simulink model "flood_drainage_system_2_R2025a"  (R2025a)
settings: Solver=VariableStepAuto  StartTime=0.0  StopTime=inf  FixedStep=1  RelTol=1e-3
undefined symbols (not defined in the file): DiscIntNeverNeededParam
libraries: simulink x15
(part 2 of 3)

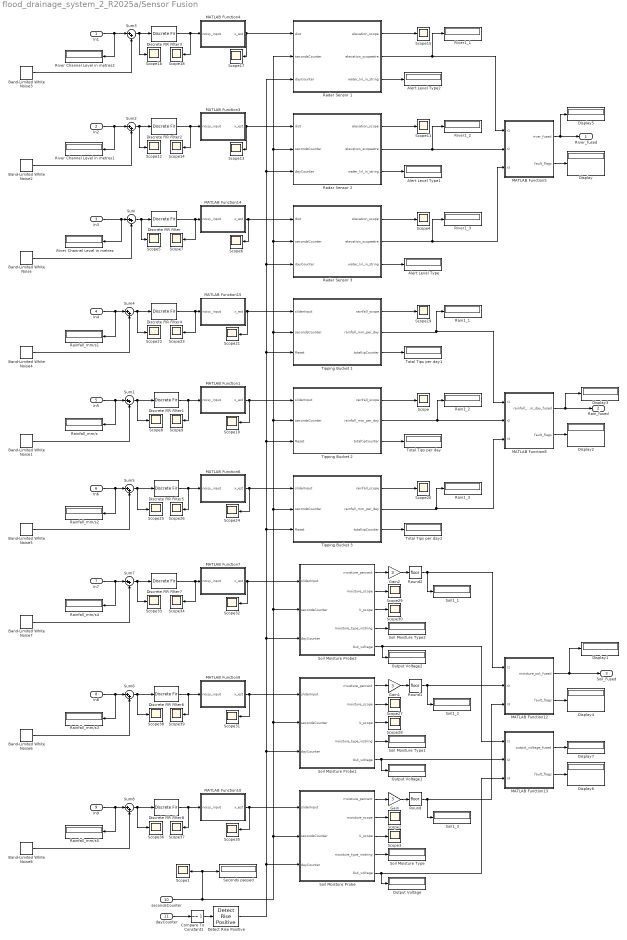
== system flood_drainage_system_2_R2025a/Sensor Fusion ==
  In1 : Inport
  In2 : Inport  Port=2
  In3 : Inport  Port=3
  In4 : Inport  Port=4
  In5 : Inport  Port=5
  In6 : Inport  Port=6
  In7 : Inport  Port=7
  In8 : Inport  Port=8
  In9 : Inport  Port=9
  secondsCounter : Inport  Port=10
  dayCounter : Inport  Port=11
  Alert Level Type : Display
  Alert Level Type1 : Display
  Alert Level Type2 : Display
  Band-Limited White Noise{,1..8} (9 alike) : simulink/Sources/Band-Limited White Noise  Cov=0.0005  Ts=1  seed=[12345]
  Compare To Constant1 : simulink/Logic and Bit Operations/Compare To Constant  relop===  const=1  OutDataTypeStr=boolean
  Detect Rise Positive : simulink/Logic and Bit Operations/Detect Rise Positive  vinit=0  OutDataTypeStr=boolean
  Discrete FIR Filter : DiscreteFir  Coefficients=[0.1 0.1 0.1 0.1 0.1 0.1 0.1 0.1 0.1 0.1]
  Discrete FIR Filter{1,4..8} (6 alike) : DiscreteFir
  Discrete FIR Filter2 : DiscreteFir  Coefficients=[0.1 0.1 0.1 0.1 0.1 0.1 0.1 0.1 0.1 0.1]
  Discrete FIR Filter3 : DiscreteFir  Coefficients=[0.1 0.1 0.1 0.1 0.1 0.1 0.1 0.1 0.1 0.1]
  Display{,1..7} (8 alike) : Display
  Gain : Gain  Gain=3
  Gain1 : Gain  Gain=3
  Gain2 : Gain  Gain=3
  MATLAB Function1 : MATLAB Function  TreatAsAtomicUnit=on
  MATLAB Function10 : MATLAB Function  TreatAsAtomicUnit=on
  MATLAB Function12 : MATLAB Function  TreatAsAtomicUnit=on
  MATLAB Function13 : MATLAB Function  TreatAsAtomicUnit=on
  MATLAB Function14 : MATLAB Function  TreatAsAtomicUnit=on
  MATLAB Function15 : MATLAB Function  TreatAsAtomicUnit=on
  MATLAB Function3 : MATLAB Function  TreatAsAtomicUnit=on
  MATLAB Function4 : MATLAB Function  TreatAsAtomicUnit=on
  MATLAB Function5 : MATLAB Function  TreatAsAtomicUnit=on
  MATLAB Function6 : MATLAB Function  TreatAsAtomicUnit=on
  MATLAB Function7 : MATLAB Function  TreatAsAtomicUnit=on
  MATLAB Function8 : MATLAB Function  TreatAsAtomicUnit=on
  MATLAB Function9 : MATLAB Function  TreatAsAtomicUnit=on
  Output Voltage : Display
  Output Voltage1 : Display
  Output Voltage2 : Display
  Radar Sensor 1 : MATLAB Function  TreatAsAtomicUnit=on
  Radar Sensor 2 : MATLAB Function  TreatAsAtomicUnit=on
  Radar Sensor 3 : MATLAB Function  TreatAsAtomicUnit=on
  Rain1_1 : Display
  Rain1_2 : Display
  Rain1_3 : Display
  Rainfall_mm/s{,1..5} (6 alike) : Display
  River Channel Level in metres : Display
  River Channel Level in metres1 : Display
  River Channel Level in metres2 : Display
  River1_1 : Display
  River1_2 : Display
  River1_3 : Display
  Round : Rounding
  Round1 : Rounding
  Round2 : Rounding
  Scope{,1..39} (40 alike) : Scope
      Scope settings: ActiveDisplayYMinimum=-10.225  ActiveDisplayYMaximum=92.025
      Scope1 settings: ActiveDisplayYMinimum=-10799.875  ActiveDisplayYMaximum=97198.875  DataLoggingVariableName=ScopeData22
      Scope10 settings: ActiveDisplayYMinimum=-0.04719  ActiveDisplayYMaximum=0.05304  DataLoggingVariableName=ScopeData23
      Scope11 settings: ActiveDisplayYMinimum=1.66242  ActiveDisplayYMaximum=5.03549  DataLoggingVariableName=ScopeData24
      Scope12 settings: ActiveDisplayYMinimum=2.1151552868576307  ActiveDisplayYMaximum=4.4405053956462046  DataLoggingVariableName=ScopeData25
      Scope13 settings: ActiveDisplayYMinimum=-1  ActiveDisplayYMaximum=1  DataLoggingVariableName=ScopeData26
      Scope14 settings: ActiveDisplayYMinimum=-1  ActiveDisplayYMaximum=1  DataLoggingVariableName=ScopeData27
      Scope15 settings: ActiveDisplayYMinimum=1.11854  ActiveDisplayYMaximum=5.0416  DataLoggingVariableName=ScopeData28
      Scope16 settings: ActiveDisplayYMinimum=3.01528  ActiveDisplayYMaximum=3.9355  DataLoggingVariableName=ScopeData29
      Scope17 settings: ActiveDisplayYMinimum=-0.04078  ActiveDisplayYMaximum=3.46295  DataLoggingVariableName=ScopeData30
      Scope18 settings: ActiveDisplayYMinimum=-0.04802  ActiveDisplayYMaximum=4.10586  DataLoggingVariableName=ScopeData31
      Scope19 settings: ActiveDisplayYMinimum=-10.225  ActiveDisplayYMaximum=92.025  DataLoggingVariableName=ScopeData32
      Scope2 settings: ActiveDisplayYMinimum=-2.30563  ActiveDisplayYMaximum=20.77423  DataLoggingVariableName=ScopeData33
      Scope20 settings: ActiveDisplayYMinimum=-10.225  ActiveDisplayYMaximum=92.025  DataLoggingVariableName=ScopeData34
      Scope21 settings: ActiveDisplayYMinimum=-0.04719  ActiveDisplayYMaximum=0.05304  DataLoggingVariableName=ScopeData35
      Scope22 settings: ActiveDisplayYMinimum=-0.13163  ActiveDisplayYMaximum=0.12145  DataLoggingVariableName=ScopeData36
      Scope23 settings: ActiveDisplayYMinimum=-0.08478  ActiveDisplayYMaximum=0.09119  DataLoggingVariableName=ScopeData5
      Scope24 settings: ActiveDisplayYMinimum=-0.04719  ActiveDisplayYMaximum=0.05304  DataLoggingVariableName=ScopeData6
      Scope25 settings: ActiveDisplayYMinimum=-0.13163  ActiveDisplayYMaximum=0.12145  DataLoggingVariableName=ScopeData7
      Scope26 settings: ActiveDisplayYMinimum=-0.08478  ActiveDisplayYMaximum=0.09119  DataLoggingVariableName=ScopeData8
      Scope27 settings: ActiveDisplayYMinimum=-3.28394  ActiveDisplayYMaximum=29.57922  DataLoggingVariableName=ScopeData9
      Scope28 settings: ActiveDisplayYMinimum=0.47959  ActiveDisplayYMaximum=0.68376  DataLoggingVariableName=ScopeData10
      Scope29 settings: ActiveDisplayYMinimum=-2.30563  ActiveDisplayYMaximum=20.77423  DataLoggingVariableName=ScopeData11
      Scope3 settings: ActiveDisplayYMinimum=0.47959  ActiveDisplayYMaximum=0.68376  DataLoggingVariableName=ScopeData37
      Scope30 settings: ActiveDisplayYMinimum=0.47959  ActiveDisplayYMaximum=0.68376  DataLoggingVariableName=ScopeData12
      Scope31 settings: ActiveDisplayYMinimum=-0.04719  ActiveDisplayYMaximum=0.05304  DataLoggingVariableName=ScopeData13
      Scope32 settings: ActiveDisplayYMinimum=-0.04719  ActiveDisplayYMaximum=0.05304  DataLoggingVariableName=ScopeData14
      Scope33 settings: ActiveDisplayYMinimum=-0.13163  ActiveDisplayYMaximum=0.12145  DataLoggingVariableName=ScopeData15
      Scope34 settings: ActiveDisplayYMinimum=-0.08478  ActiveDisplayYMaximum=0.09119  DataLoggingVariableName=ScopeData16
      Scope35 settings: ActiveDisplayYMinimum=-0.04719  ActiveDisplayYMaximum=0.05304  DataLoggingVariableName=ScopeData17
      Scope36 settings: ActiveDisplayYMinimum=-0.13163  ActiveDisplayYMaximum=0.12145  DataLoggingVariableName=ScopeData18
      Scope37 settings: ActiveDisplayYMinimum=-0.08478  ActiveDisplayYMaximum=0.09119  DataLoggingVariableName=ScopeData19
      Scope38 settings: ActiveDisplayYMinimum=-0.13163  ActiveDisplayYMaximum=0.12145  DataLoggingVariableName=ScopeData20
      Scope39 settings: ActiveDisplayYMinimum=-0.08478  ActiveDisplayYMaximum=0.09119  DataLoggingVariableName=ScopeData21
      Scope4 settings: ActiveDisplayYMinimum=2.19395  ActiveDisplayYMaximum=5.02952  DataLoggingVariableName=ScopeData4
      Scope5 settings: ActiveDisplayYMinimum=3.01528  ActiveDisplayYMaximum=3.9355  DataLoggingVariableName=ScopeData38
      Scope6 settings: ActiveDisplayYMinimum=-0.03897  ActiveDisplayYMaximum=3.3021  DataLoggingVariableName=ScopeData39
      Scope7 settings: ActiveDisplayYMinimum=-0.03899  ActiveDisplayYMaximum=3.30223  DataLoggingVariableName=ScopeData3
      Scope8 settings: ActiveDisplayYMinimum=-0.13163  ActiveDisplayYMaximum=0.12145
      Scope9 settings: ActiveDisplayYMinimum=-0.08478  ActiveDisplayYMaximum=0.09119  DataLoggingVariableName=ScopeData2
  Seconds passed : Display
  Soil Moisture Probe : MATLAB Function  TreatAsAtomicUnit=on
  Soil Moisture Probe1 : MATLAB Function  TreatAsAtomicUnit=on
  Soil Moisture Probe2 : MATLAB Function  TreatAsAtomicUnit=on
  Soil Moisture Type : Display
  Soil Moisture Type1 : Display
  Soil Moisture Type2 : Display
  Soil1_1 : Display
  Soil1_2 : Display
  Soil1_3 : Display
  Sum{,1..8} (9 alike) : Sum  Inputs=|++
  Tipping Bucket 1 : Stateflow chart  TreatAsAtomicUnit=on
      settings: PortSchema="{\"entries\":[{\"content\":{\"sides\":[{\"content\":{\"connectorIds\":[\"In1\",\"In2\",\"In3\"]},\"type\":\"ConnectorPlacement.EquallySpacedRectSide\",\"uuid\":\"5446b20b-2648-415f-9f86-c4722c72a7ab\"},{\"content\":{\"connectorIds\":[\"Out2\",\"Out3\",\"Out1\"],\"side\":\"RIGHT\"},\"type\":\"ConnectorPlacement.EquallySpacedRectSide\",\"uuid\":\"249dbc32-ec03-48ca-bf45-e180eac5a0e9\"},{\"content\":{\"side\":\"TOP\"},\"type\":\"ConnectorPlacement.EquallySpacedRectSide\",\"uuid\":\"c4af4b86-9bbe-4324-913f-65d0095b4577\"}]},\"type\":\"ConnectorPlacement.EquallySpacedConnector\",\"uuid\":\"ebffaa42-42d2-45af-8401-087243cf8eee\"}],\"packageUris\":[\"http://schema.mathworks.com/mf0/Connector/R2020b\"],\"version\":\"1.0\"}"
  Tipping Bucket 2 : Stateflow chart  TreatAsAtomicUnit=on
      settings: PortSchema="{\"entries\":[{\"content\":{\"sides\":[{\"content\":{\"connectorIds\":[\"In1\",\"In2\",\"In3\"]},\"type\":\"ConnectorPlacement.EquallySpacedRectSide\",\"uuid\":\"5446b20b-2648-415f-9f86-c4722c72a7ab\"},{\"content\":{\"connectorIds\":[\"Out2\",\"Out3\",\"Out1\"],\"side\":\"RIGHT\"},\"type\":\"ConnectorPlacement.EquallySpacedRectSide\",\"uuid\":\"249dbc32-ec03-48ca-bf45-e180eac5a0e9\"},{\"content\":{\"side\":\"TOP\"},\"type\":\"ConnectorPlacement.EquallySpacedRectSide\",\"uuid\":\"c4af4b86-9bbe-4324-913f-65d0095b4577\"}]},\"type\":\"ConnectorPlacement.EquallySpacedConnector\",\"uuid\":\"ebffaa42-42d2-45af-8401-087243cf8eee\"}],\"packageUris\":[\"http://schema.mathworks.com/mf0/Connector/R2020b\"],\"version\":\"1.0\"}"
  Tipping Bucket 3 : Stateflow chart  TreatAsAtomicUnit=on
      settings: PortSchema="{\"entries\":[{\"content\":{\"sides\":[{\"content\":{\"connectorIds\":[\"In1\",\"In2\",\"In3\"]},\"type\":\"ConnectorPlacement.EquallySpacedRectSide\",\"uuid\":\"5446b20b-2648-415f-9f86-c4722c72a7ab\"},{\"content\":{\"connectorIds\":[\"Out2\",\"Out3\",\"Out1\"],\"side\":\"RIGHT\"},\"type\":\"ConnectorPlacement.EquallySpacedRectSide\",\"uuid\":\"249dbc32-ec03-48ca-bf45-e180eac5a0e9\"},{\"content\":{\"side\":\"TOP\"},\"type\":\"ConnectorPlacement.EquallySpacedRectSide\",\"uuid\":\"c4af4b86-9bbe-4324-913f-65d0095b4577\"}]},\"type\":\"ConnectorPlacement.EquallySpacedConnector\",\"uuid\":\"ebffaa42-42d2-45af-8401-087243cf8eee\"}],\"packageUris\":[\"http://schema.mathworks.com/mf0/Connector/R2020b\"],\"version\":\"1.0\"}"
  Total Tips per day : Display
  Total Tips per day1 : Display
  Total Tips per day2 : Display
  River_fused : Outport
  Rain_fused : Outport  Port=2
  Soil_Fused : Outport  Port=3
  wires:
  Tipping Bucket 1/1(totaltipCounter) -> Total Tips per day1/1
  MATLAB Function14/1(x_est) -> Scope6/1, Radar Sensor 3/1(dist)
  Soil Moisture Probe/4(moisture_type_instring) -> Soil Moisture Type/1
  Tipping Bucket 2/3(rainfall_mm_per_day) -> MATLAB Function8/2(r2), Rain1_2/1
  MATLAB Function6/1(x_est) -> Scope24/1, Tipping Bucket 3/1(sliderInput)
  Soil Moisture Probe2/5(Out_voltage) -> MATLAB Function13/1(r1), Output Voltage2/1
  MATLAB Function13/2(fault_flags) -> Display6/1
  Sum2/1 -> Discrete FIR Filter2/1, Scope12/1
  Discrete FIR Filter8/1 -> MATLAB Function10/1(noisy_input), Scope37/1
  Discrete FIR Filter7/1 -> MATLAB Function7/1(noisy_input), Scope34/1
  Sum/1 -> Discrete FIR Filter/1, Scope5/1
  MATLAB Function8/2(fault_flags) -> Display2/1
  Tipping Bucket 3/1(totaltipCounter) -> Total Tips per day2/1
  In3/1 -> Sum/1, River Channel Level in metres/1
  Discrete FIR Filter1/1 -> MATLAB Function1/1(noisy_input), Scope9/1
  Soil Moisture Probe/1(moisture_percent) -> Gain/1
  MATLAB Function10/1(x_est) -> Soil Moisture Probe/1(sliderInput), Scope35/1
  Band-Limited White Noise5/1 -> Sum5/2
  Band-Limited White Noise8/1 -> Sum8/2
  Radar Sensor 2/1(elevation_scope) -> Scope11/1
  Sum7/1 -> Scope33/1, Discrete FIR Filter7/1
  In7/1 -> Sum7/1, Rainfall_mm/s4/1
  MATLAB Function7/1(x_est) -> Soil Moisture Probe2/1(sliderInput), Scope32/1
  In4/1 -> Sum4/1, Rainfall_mm/s1/1
  Band-Limited White Noise3/1 -> Sum3/2
  Sum1/1 -> Scope8/1, Discrete FIR Filter1/1
  Gain1/1 -> Round1/1
  secondsCounter/1 -> Seconds passed/1, Scope1/1, Soil Moisture Probe1/2(secondsCounter), Soil Moisture Probe2/2(secondsCounter), Tipping Bucket 3/2(secondsCounter), Tipping Bucket 1/2(secondsCounter), Radar Sensor 1/2(secondsCounter), Radar Sensor 2/2(secondsCounter), Radar Sensor 3/2(secondsCounter), Tipping Bucket 2/2(secondsCounter), Soil Moisture Probe/2(secondsCounter)
  Tipping Bucket 1/3(rainfall_mm_per_day) -> MATLAB Function8/1(r1), Rain1_1/1
  MATLAB Function12/2(fault_flags) -> Display4/1
  MATLAB Function9/1(x_est) -> Soil Moisture Probe1/1(sliderInput), Scope31/1
  Tipping Bucket 3/3(rainfall_mm_per_day) -> MATLAB Function8/3(r3), Rain1_3/1
  Soil Moisture Probe2/3(V_scope) -> Scope30/1
  Discrete FIR Filter6/1 -> MATLAB Function9/1(noisy_input), Scope39/1
  MATLAB Function1/1(x_est) -> Scope10/1, Tipping Bucket 2/1(sliderInput)
  Soil Moisture Probe/5(Out_voltage) -> MATLAB Function13/3(r3), Output Voltage/1
  Band-Limited White Noise/1 -> Sum/2
  Radar Sensor 1/1(elevation_scope) -> Scope15/1
  In6/1 -> Sum5/1, Rainfall_mm/s2/1
  In5/1 -> Sum1/1, Rainfall_mm/s/1
  Sum8/1 -> Scope36/1, Discrete FIR Filter8/1
  MATLAB Function8/1(rainfall_mm_day_fused) -> Display3/1, Rain_fused/1
  Radar Sensor 3/1(elevation_scope) -> Scope4/1
  Sum4/1 -> Scope22/1, Discrete FIR Filter4/1
  Tipping Bucket 2/1(totaltipCounter) -> Total Tips per day/1
  In2/1 -> Sum2/1, River Channel Level in metres1/1
  Discrete FIR Filter5/1 -> MATLAB Function6/1(noisy_input), Scope26/1
  Round1/1 -> MATLAB Function12/2(r2), Soil1_2/1
  MATLAB Function13/1(output_voltage_fused) -> Display7/1
  Radar Sensor 1/2(elevation_scopeetre) -> MATLAB Function5/1(r1), River1_1/1
  MATLAB Function4/1(x_est) -> Radar Sensor 1/1(dist), Scope17/1
  Discrete FIR Filter/1 -> Scope7/1, MATLAB Function14/1(noisy_input)
  Compare To Constant1/1 -> Detect Rise Positive/1
  Discrete FIR Filter4/1 -> MATLAB Function15/1(noisy_input), Scope23/1
  Band-Limited White Noise2/1 -> Sum2/2
  Radar Sensor 3/2(elevation_scopeetre) -> MATLAB Function5/3(r3), River1_3/1
  Round/1 -> Soil1_3/1, MATLAB Function12/3(r3)
  Detect Rise Positive/1 -> Soil Moisture Probe1/3(dayCounter), Soil Moisture Probe2/3(dayCounter), Tipping Bucket 3/3(Reset), Tipping Bucket 1/3(Reset), Radar Sensor 1/3(dayCounter), Radar Sensor 2/3(dayCounter), Radar Sensor 3/3(dayCounter), Tipping Bucket 2/3(Reset), Soil Moisture Probe/3(dayCounter)
  MATLAB Function15/1(x_est) -> Scope21/1, Tipping Bucket 1/1(sliderInput)
  Sum3/1 -> Discrete FIR Filter3/1, Scope16/1
  In8/1 -> Sum6/1, Rainfall_mm/s3/1
  Gain/1 -> Round/1
  MATLAB Function5/1(river_fused) -> Display5/1, River_fused/1
  Soil Moisture Probe1/2(moisture_scope) -> Scope27/1
  Discrete FIR Filter3/1 -> Scope18/1, MATLAB Function4/1(noisy_input)
  Soil Moisture Probe2/4(moisture_type_instring) -> Soil Moisture Type2/1
  Radar Sensor 3/3(water_lvl_in_string) -> Alert Level Type/1
  MATLAB Function3/1(x_est) -> Radar Sensor 2/1(dist), Scope13/1
  Sum6/1 -> Scope38/1, Discrete FIR Filter6/1
  Soil Moisture Probe1/3(V_scope) -> Scope28/1
  Soil Moisture Probe/3(V_scope) -> Scope3/1
  Tipping Bucket 1/2(rainfall_scope) -> Scope19/1
  Band-Limited White Noise4/1 -> Sum4/2
  Discrete FIR Filter2/1 -> MATLAB Function3/1(noisy_input), Scope14/1
  Band-Limited White Noise7/1 -> Sum7/2
  Round2/1 -> MATLAB Function12/1(r1), Soil1_1/1
  MATLAB Function5/2(fault_flags) -> Display/1
  Gain2/1 -> Round2/1
  Soil Moisture Probe2/1(moisture_percent) -> Gain2/1
  Tipping Bucket 2/2(rainfall_scope) -> Scope/1
  Radar Sensor 2/3(water_lvl_in_string) -> Alert Level Type1/1
  Soil Moisture Probe2/2(moisture_scope) -> Scope29/1
  In9/1 -> Sum8/1, Rainfall_mm/s5/1
  Soil Moisture Probe1/1(moisture_percent) -> Gain1/1
  Radar Sensor 2/2(elevation_scopeetre) -> River1_2/1, MATLAB Function5/2(r2)
  Soil Moisture Probe/2(moisture_scope) -> Scope2/1
  Sum5/1 -> Scope25/1, Discrete FIR Filter5/1
  Radar Sensor 1/3(water_lvl_in_string) -> Alert Level Type2/1
  Band-Limited White Noise6/1 -> Sum6/2
  Band-Limited White Noise1/1 -> Sum1/2
  Soil Moisture Probe1/5(Out_voltage) -> MATLAB Function13/2(r2), Output Voltage1/1
  Soil Moisture Probe1/4(moisture_type_instring) -> Soil Moisture Type1/1
  In1/1 -> Sum3/1, River Channel Level in metres2/1
  MATLAB Function12/1(moisture_pct_fused) -> Display1/1, Soil_Fused/1
  Tipping Bucket 3/2(rainfall_scope) -> Scope20/1
  dayCounter/1 -> Compare To Constant1/1

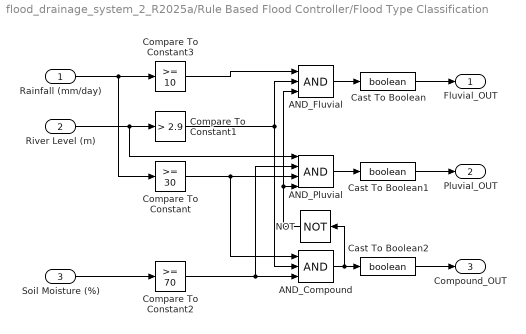
== system flood_drainage_system_2_R2025a/Rule Based Flood Controller/Flood Type Classification ==
  Rainfall (mm/day) : Inport
  River Level (m) : Inport  Port=2
  Soil Moisture (%) : Inport  Port=3
  AND_Compound : Logic  Inputs=3  IconShape=distinctive  AllPortsSameDT=off  OutDataTypeStr=boolean
  AND_Fluvial : Logic  Inputs=3  IconShape=distinctive  AllPortsSameDT=off  OutDataTypeStr=boolean
  AND_Pluvial : Logic  Inputs=4  IconShape=distinctive  AllPortsSameDT=off  OutDataTypeStr=boolean
  Cast To Boolean : DataTypeConversion  OutDataTypeStr=boolean  SaturateOnIntegerOverflow=off  RndMeth=Floor
  Cast To Boolean1 : DataTypeConversion  OutDataTypeStr=boolean  SaturateOnIntegerOverflow=off  RndMeth=Floor
  Cast To Boolean2 : DataTypeConversion  OutDataTypeStr=boolean  SaturateOnIntegerOverflow=off  RndMeth=Floor
  Compare To Constant : simulink/Logic and Bit Operations/Compare To Constant  relop=>=  const=30  OutDataTypeStr=boolean
  Compare To Constant1 : simulink/Logic and Bit Operations/Compare To Constant  relop=>  const=2.9  OutDataTypeStr=boolean
  Compare To Constant2 : simulink/Logic and Bit Operations/Compare To Constant  relop=>=  const=70  OutDataTypeStr=boolean
  Compare To Constant3 : simulink/Logic and Bit Operations/Compare To Constant  relop=>=  const=10  OutDataTypeStr=boolean
  NOT : Logic  Operator=NOT  IconShape=distinctive  AllPortsSameDT=off  OutDataTypeStr=boolean
  Fluvial_OUT : Outport
  Pluvial_OUT : Outport  Port=2
  Compound_OUT : Outport  Port=3
  wires:
  Rainfall (mm/day)/1 -> Compare To Constant/1, Compare To Constant3/1
  River Level (m)/1 -> AND_Pluvial/1, Compare To Constant1/1
  Soil Moisture (%)/1 -> Compare To Constant2/1
  Compare To Constant/1 -> AND_Compound/1, AND_Pluvial/3
  Compare To Constant1/1 -> AND_Fluvial/2, AND_Compound/2
  Compare To Constant2/1 -> AND_Pluvial/2, AND_Compound/3
  Compare To Constant3/1 -> AND_Fluvial/1
  AND_Fluvial/1 -> Cast To Boolean/1
  Cast To Boolean/1 -> Fluvial_OUT/1
  Cast To Boolean1/1 -> Pluvial_OUT/1
  AND_Compound/1 -> NOT/1, Cast To Boolean2/1
  AND_Pluvial/1 -> Cast To Boolean1/1
  Cast To Boolean2/1 -> Compound_OUT/1
  NOT/1 -> AND_Fluvial/3, AND_Pluvial/4

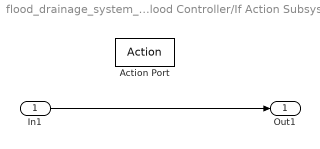
== system flood_drainage_system_2_R2025a/Rule Based Flood Controller/If Action Subsystem ==
  In1 : Inport
  Action Port : ActionPort  ActionPortLabel=if(u1 <= 0.3)
  Out1 : Outport
  wires:
  In1/1 -> Out1/1

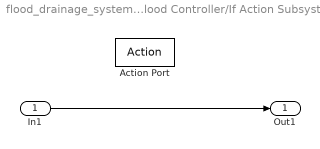
== system flood_drainage_system_2_R2025a/Rule Based Flood Controller/If Action Subsystem1 ==
  In1 : Inport
  Action Port : ActionPort  ActionPortLabel=elseif(u1 <= 0.6)
  Out1 : Outport
  wires:
  In1/1 -> Out1/1

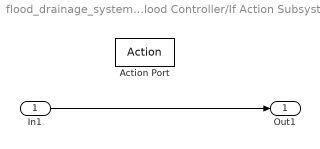
== system flood_drainage_system_2_R2025a/Rule Based Flood Controller/If Action Subsystem2 ==
  In1 : Inport
  Action Port : ActionPort  ActionPortLabel=elseif(u1 < 0.8)
  Out1 : Outport
  wires:
  In1/1 -> Out1/1

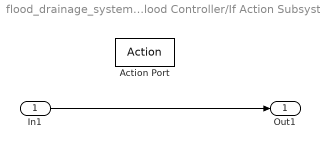
== system flood_drainage_system_2_R2025a/Rule Based Flood Controller/If Action Subsystem3 ==
  In1 : Inport
  Action Port : ActionPort  ActionPortLabel=else
  Out1 : Outport
  wires:
  In1/1 -> Out1/1

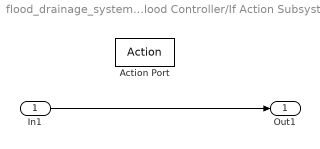
== system flood_drainage_system_2_R2025a/Rule Based Flood Controller/If Action Subsystem4 ==
  In1 : Inport
  Action Port : ActionPort  ActionPortLabel=if(u1==1)
  Out1 : Outport
  wires:
  In1/1 -> Out1/1

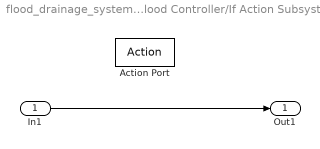
== system flood_drainage_system_2_R2025a/Rule Based Flood Controller/If Action Subsystem5 ==
  In1 : Inport
  Action Port : ActionPort  ActionPortLabel=elseif(u1==2)
  Out1 : Outport
  wires:
  In1/1 -> Out1/1

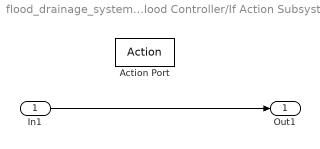
== system flood_drainage_system_2_R2025a/Rule Based Flood Controller/If Action Subsystem6 ==
  In1 : Inport
  Action Port : ActionPort  ActionPortLabel=elseif(u1==3)
  Out1 : Outport
  wires:
  In1/1 -> Out1/1

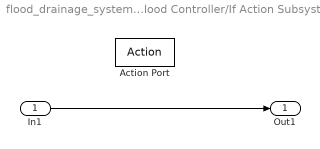
== system flood_drainage_system_2_R2025a/Rule Based Flood Controller/If Action Subsystem7 ==
  In1 : Inport
  Action Port : ActionPort  ActionPortLabel=else
  Out1 : Outport
  wires:
  In1/1 -> Out1/1

== matlab function flood_drainage_system_2_R2025a/Sensor Fusion/Radar Sensor 2 ==
  data: dist input; elevation_scope output; secondsCounter input; dayCounter input; elevation_scopeetre output; water_lvl_in_string output
function [elevation_scope, elevation_scopeetre, water_lvl_in_string] = ...
          riverElevationSensor(dist, secondsCounter, dayCounter)

ref_elev = 5.0; % reference elevation (m)

persistent prevSec prevDay elevation elevation_last water_lvl_code_last water_lvl_str_last
if isempty(prevSec), prevSec = 0; end
if isempty(prevDay), prevDay = 0; end
if isempty(elevation), elevation = ref_elev - dist; end
if isempty(elevation_last), elevation_last = ref_elev - dist; end
if isempty(water_lvl_code_last), water_lvl_code_last = 0; end
if isempty(water_lvl_str_last), water_lvl_str_last = "Error"; end

deltaT = secondsCounter - prevSec;
if deltaT <= 0
    deltaT = 1;
end

% update elevation by the second
target_elev = ref_elev - dist;
rate = (target_elev - elevation) / 1000; % smoothing factor
elevation = elevation + rate * deltaT;

% classification
% If elevation_scope is higher than:
% 1.7 m = Critical
% 2.05 m = Alert
% 2.2 m = Normal

if elevation > 2.05 % Below 2.05 m = Normal
    water_lvl_code = 1; % Normal
    water_lvl_str = "Normal";
elseif (elevation <= 2.05 && elevation > 1.7)
    water_lvl_code = 2; % Alert
    water_lvl_str = "Alert";
elseif elevation <= 1.7 
    water_lvl_code = 3; % Critical
    water_lvl_str = "Critical";
else
    water_lvl_code = 0; % Error
    water_lvl_str = "Error";
end

% reset logic
if double(dayCounter) ~= double(prevDay)
    elevation_last = elevation;
    water_lvl_code_last = water_lvl_code;
    water_lvl_str_last = water_lvl_str;
    prevDay = double(dayCounter);
end

% update state
prevSec = secondsCounter;

% outputs
elevation_scope = elevation;
elevation_scopeetre = elevation_last;
water_lvl_in_string = water_lvl_str_last;

== matlab function flood_drainage_system_2_R2025a/MATLAB Function2 ==
  data: secondsCounter output; dayCounter output; u input
function [secondsCounter, dayCounter] = timerFcn(u)

persistent seconds day
if isempty(seconds)
    seconds = 0;
end

if isempty(day)
    day = 0;
end

% count seconds to full day
seconds = seconds + 1;

% full day passed (24 hours = 86400 sec)
if mod(seconds,86400 ) == 0
    day = day + 1;
end

% output
secondsCounter = mod(seconds,86400);
dayCounter = day;

== matlab function flood_drainage_system_2_R2025a/Sensor Fusion/Soil Moisture Probe ==
  data: moisture_percent output; moisture_scope output; V_scope output; sliderInput input; secondsCounter input; dayCounter input; moisture_type_instring output; Out_voltage output
function [moisture_percent, moisture_scope, V_scope, moisture_type_instring, Out_voltage] = ...
          soilMoistureProbe(sliderInput, secondsCounter, dayCounter)

infil_eff = 0.7;       % infiltration efficiency
d = 300;               % soil depth (mm)
ET_day = 2;            % evapotranspiration loss (mm/day)
ET_rate = ET_day / 86400; % mm/s

persistent VWC prevSec prevDay moisture_scope_last moisture_type_last V_scope_last
if isempty(VWC), VWC = 0; end
if isempty(prevSec), prevSec = 0; end
if isempty(prevDay), prevDay = 0; end
if isempty(moisture_scope_last), moisture_scope_last = 0; end
if isempty(moisture_type_last), moisture_type_last = ""; end
if isempty(V_scope_last), V_scope_last = 0; end

% deltaT (seconds since last tick)
deltaT = secondsCounter - prevSec;
if deltaT <= 0
    deltaT = 1;
end

% rainfall over deltaT (per sec)
rain_mm = sliderInput * deltaT;          % mm of rain in deltaT (per sec)
infil_mm = infil_eff * rain_mm;          % effective infiltration
rain_frac = infil_mm / d;                % fraction of saturation

% ET contribution over deltaT
ET_mm = ET_rate * deltaT;                % mm lost in deltaT
ET_frac = ET_mm / d;                     % fraction of saturation

% Update cumulative Volume Water Concentration (VWC) in fraction
VWC = VWC + rain_frac - ET_frac;
moisture_scope = VWC * 100;

% keep between 0 to 100 only
moisture_scope = max(0, min(100, moisture_scope));
VWC = moisture_scope / 100; 

% classification
if  moisture_scope < 10 % 30
    moisture_type = "Dry";
elseif moisture_scope < 20 % 60
    moisture_type = "Moderate";
elseif moisture_scope < 30 % 90
    moisture_type = "Wet";
else
    moisture_type = "Saturated";
end

% voltage output
V_scope = 0.5 + (moisture_scope/100);

% reset logic (daily rollover)
if double(dayCounter) ~= double(prevDay)
    moisture_scope_last = moisture_scope;
    moisture_type_last = moisture_type;
    V_scope_last = V_scope;

    % carry forward baseline
    VWC = moisture_scope / 100;
    prevDay = double(dayCounter);
end

% update state
prevSec = secondsCounter;

% outputs
moisture_percent = moisture_scope_last;
moisture_type_instring = moisture_type_last;
Out_voltage = V_scope_last;

== matlab function flood_drainage_system_2_R2025a/Sensor Fusion/Radar Sensor 3 ==
  data: dist input; elevation_scope output; secondsCounter input; dayCounter input; elevation_scopeetre output; water_lvl_in_string output
function [elevation_scope, elevation_scopeetre, water_lvl_in_string] = ...
          riverElevationSensor(dist, secondsCounter, dayCounter)

ref_elev = 5.0; % reference elevation (m)

persistent prevSec prevDay elevation elevation_last water_lvl_code_last water_lvl_str_last
if isempty(prevSec), prevSec = 0; end
if isempty(prevDay), prevDay = 0; end
if isempty(elevation), elevation = ref_elev - dist; end
if isempty(elevation_last), elevation_last = ref_elev - dist; end
if isempty(water_lvl_code_last), water_lvl_code_last = 0; end
if isempty(water_lvl_str_last), water_lvl_str_last = "Error"; end

deltaT = secondsCounter - prevSec;
if deltaT <= 0
    deltaT = 1;
end

% update elevation by the second
target_elev = ref_elev - dist;
rate = (target_elev - elevation) / 1000; % smoothing factor
elevation = elevation + rate * deltaT;

% classification
% If elevation_scope is higher than:
% 1.7 m = Critical
% 2.05 m = Alert
% 2.2 m = Normal

if elevation > 2.05 % Below 2.05 m = Normal
    water_lvl_code = 1; % Normal
    water_lvl_str = "Normal";
elseif (elevation <= 2.05 && elevation > 1.7)
    water_lvl_code = 2; % Alert
    water_lvl_str = "Alert";
elseif elevation <= 1.7 
    water_lvl_code = 3; % Critical
    water_lvl_str = "Critical";
else
    water_lvl_code = 0; % Error
    water_lvl_str = "Error";
end

% reset logic
if double(dayCounter) ~= double(prevDay)
    elevation_last = elevation;
    water_lvl_code_last = water_lvl_code;
    water_lvl_str_last = water_lvl_str;
    prevDay = double(dayCounter);
end

% update state
prevSec = secondsCounter;

% outputs
elevation_scope = elevation;
elevation_scopeetre = elevation_last;
water_lvl_in_string = water_lvl_str_last;

== matlab function flood_drainage_system_2_R2025a/Sensor Fusion/MATLAB Function4 ==
  data: noisy_input input; x_est output
function x_est = kalmanFilter(noisy_input)

persistent x P
if isempty(x), x = noisy_input; end
if isempty(P), P = 1; end


Q = 1e-3;   % process noise covariance
R = 1e-4;   % measurement noise covariance

% prediction
x_pred = x;
P_pred = P + Q;

% update
K = P_pred / (P_pred + R);
x = x_pred + K*(noisy_input - x_pred);
P = (1 - K)*P_pred;

x_est = x;

== matlab function flood_drainage_system_2_R2025a/Sensor Fusion/Radar Sensor 1 ==
  data: dist input; elevation_scope output; secondsCounter input; dayCounter input; elevation_scopeetre output; water_lvl_in_string output
function [elevation_scope, elevation_scopeetre, water_lvl_in_string] = ...
          riverElevationSensor(dist, secondsCounter, dayCounter)

ref_elev = 5.0; % reference elevation (m)

persistent prevSec prevDay elevation elevation_last water_lvl_code_last water_lvl_str_last
if isempty(prevSec), prevSec = 0; end
if isempty(prevDay), prevDay = 0; end
if isempty(elevation), elevation = ref_elev - dist; end
if isempty(elevation_last), elevation_last = ref_elev - dist; end
if isempty(water_lvl_code_last), water_lvl_code_last = 0; end
if isempty(water_lvl_str_last), water_lvl_str_last = "Error"; end

deltaT = secondsCounter - prevSec;
if deltaT <= 0
    deltaT = 1;
end

% update elevation by the second
target_elev = ref_elev - dist;
rate = (target_elev - elevation) / 1000; % smoothing factor
elevation = elevation + rate * deltaT;

% classification
% If elevation_scope is higher than:
% 1.7 m = Critical
% 2.05 m = Alert
% 2.2 m = Normal

if elevation > 2.05 % Below 2.05 m = Normal
    water_lvl_code = 1; % Normal
    water_lvl_str = "Normal";
elseif (elevation <= 2.05 && elevation > 1.7)
    water_lvl_code = 2; % Alert
    water_lvl_str = "Alert";
elseif elevation <= 1.7 
    water_lvl_code = 3; % Critical
    water_lvl_str = "Critical";
else
    water_lvl_code = 0; % Error
    water_lvl_str = "Error";
end

% reset logic
if double(dayCounter) ~= double(prevDay)
    elevation_last = elevation;
    water_lvl_code_last = water_lvl_code;
    water_lvl_str_last = water_lvl_str;
    prevDay = double(dayCounter);
end

% update state
prevSec = secondsCounter;

% outputs
elevation_scope = elevation;
elevation_scopeetre = elevation_last;
water_lvl_in_string = water_lvl_str_last;

== matlab function flood_drainage_system_2_R2025a/Sensor Fusion/MATLAB Function5 ==
  data: r1 input; river_fused output; r2 input; r3 input; fault_flags output
function [river_fused, fault_flags] = fuseRiverSensors(r1, r2, r3)
% r1, r2, r3 = filtered outputs from 3 sensor chains
% river_fused = fused river elevation signal (scalar double)
% fault_flags = [f1 f2 f3], 1 if sensor flagged faulty

% Parameters
tol = 0.10; % 10% tolerance

% Step 1: Compute mean
vals = [r1 r2 r3];
mean_val = mean(vals);

% Step 2: Fault detection
fault_flags = abs(vals - mean_val) > tol*mean_val;

% Step 3: Fuse valid sensors
valid_vals = vals(~fault_flags);

if isempty(valid_vals)
    % All faulty → fallback to mean
    river_fused = mean_val;
elseif isscalar(valid_vals)
    % Only one valid → use it directly (scalar)
    river_fused = valid_vals(1);
elseif numel(valid_vals) == 2
    % Two valid → average them (scalar)
    river_fused = mean(valid_vals);
else
    % All valid (3) → use median (scalar)
    river_fused = median(valid_vals);
end

== stateflow chart flood_drainage_system_2_R2025a/Sensor Fusion/Tipping Bucket 1 ==
  state Collecting
    during:
    [accumulation, tipCounter, rainfall_scope] = bucketMath(sliderInput, secondsCounter);
  state Reset_Signal
    entry:
    rainfall_mm_per_day = rainfall_scope;
    totaltipCounter = tipCounter;
    tipCounter = 0;
    accumulation = 0;
    rainfall_scope = 0;
  (default) -> Collecting
  Reset_Signal -> Collecting
  Collecting -> Reset_Signal : [Reset == 1]
  data: sliderInput function_input; accumulation function_output; tipCounter function_output; rainfall_scope function_output; secondsCounter function_input; totaltipCounter output; rainfall_scope output; sliderInput input; accumulation local; secondsCounter input; Reset input; rainfall_mm_per_day output; tipCounter local
  function [accumulation, tipCounter, rainfall_scope] = bucketMath(sliderInput, secondsCounter):
    | function [accumulation, tipCounter, rainfall_scope] = bucketMath(sliderInput, secondsCounter)
    | 
    | persistent acc tips prevSec
    | if isempty(acc), acc = 0; end
    | if isempty(tips), tips = 0; end
    | if isempty(prevSec), prevSec = 0; end
    | 
    | deltaT = secondsCounter - prevSec;
    | if deltaT <= 0, deltaT = 1; end
    | 
    | acc = acc + sliderInput * deltaT;
    | if acc >= 0.2
    |     tips = tips + 1;
    |     acc = acc - 0.2;
    | end
    | 
    | rainfall_scope = tips * 0.2;
    | prevSec = secondsCounter;
    | 
    | accumulation = acc;
    | tipCounter = tips;

== stateflow chart flood_drainage_system_2_R2025a/Sensor Fusion/Tipping Bucket 2 ==
  state Collecting
    during:
    [accumulation, tipCounter, rainfall_scope] = bucketMath(sliderInput, secondsCounter);
  state Reset_Signal
    entry:
    rainfall_mm_per_day = rainfall_scope;
    totaltipCounter = tipCounter;
    tipCounter = 0;
    accumulation = 0;
    rainfall_scope = 0;
  (default) -> Collecting
  Reset_Signal -> Collecting
  Collecting -> Reset_Signal : [Reset == 1]
  data: sliderInput function_input; accumulation function_output; tipCounter function_output; rainfall_scope function_output; secondsCounter function_input; totaltipCounter output; rainfall_scope output; sliderInput input; accumulation local; secondsCounter input; Reset input; rainfall_mm_per_day output; tipCounter local
  function [accumulation, tipCounter, rainfall_scope] = bucketMath(sliderInput, secondsCounter):
    | function [accumulation, tipCounter, rainfall_scope] = bucketMath(sliderInput, secondsCounter)
    | persistent acc tips prevSec
    | if isempty(acc), acc = 0; end
    | if isempty(tips), tips = 0; end
    | if isempty(prevSec), prevSec = 0; end
    | 
    | deltaT = secondsCounter - prevSec;
    | if deltaT <= 0, deltaT = 1; end
    | 
    | acc = acc + sliderInput * deltaT;
    | if acc >= 0.2
    |     tips = tips + 1;
    |     acc = acc - 0.2;
    | end
    | 
    | rainfall_scope = tips * 0.2;
    | prevSec = secondsCounter;
    | 
    | accumulation = acc;
    | tipCounter = tips;

== matlab function flood_drainage_system_2_R2025a/Sensor Fusion/MATLAB Function6 ==
  data: noisy_input input; x_est output
function x_est = kalmanFilter(noisy_input)

persistent x P
if isempty(x), x = noisy_input; end
if isempty(P), P = 1; end


Q = 1e-3;   % process noise covariance
R = 1e-4;   % measurement noise covariance

% prediction
x_pred = x;
P_pred = P + Q;

% update
K = P_pred / (P_pred + R);
x = x_pred + K*(noisy_input - x_pred);
P = (1 - K)*P_pred;

x_est = x;

== matlab function flood_drainage_system_2_R2025a/Sensor Fusion/MATLAB Function7 ==
  data: noisy_input input; x_est output
function x_est = kalmanFilter(noisy_input)

persistent x P
if isempty(x), x = noisy_input; end
if isempty(P), P = 1; end


Q = 1e-3;   % process noise covariance
R = 1e-4;   % measurement noise covariance

% prediction
x_pred = x;
P_pred = P + Q;

% update
K = P_pred / (P_pred + R);
x = x_pred + K*(noisy_input - x_pred);
P = (1 - K)*P_pred;

x_est = x;

== matlab function flood_drainage_system_2_R2025a/Sensor Fusion/MATLAB Function8 ==
  data: r1 input; rainfall_mm_day_fused output; r2 input; r3 input; fault_flags output
function [rainfall_mm_day_fused, fault_flags] = fuseTipBucSensors(r1, r2, r3)
% r1, r2, r3 = filtered outputs from 3 sensor chains
% rainfall_mm_day_fused = fused river elevation signal (scalar double)
% fault_flags = [f1 f2 f3], 1 if sensor flagged faulty

% Parameters
tol = 0.15; % 15% tolerance

% Step 1: Compute mean
vals = [r1 r2 r3];
mean_val = mean(vals);

% Step 2: Fault detection
fault_flags = abs(vals - mean_val) > tol*mean_val;

% Step 3: Fuse valid sensors
valid_vals = vals(~fault_flags);

if isempty(valid_vals)
    % All faulty → fallback to mean
    rainfall_mm_day_fused = mean_val;
elseif isscalar(valid_vals)
    % Only one valid → use it directly (scalar)
    rainfall_mm_day_fused = valid_vals(1);
elseif numel(valid_vals) == 2
    % Two valid → average them (scalar)
    rainfall_mm_day_fused = mean(valid_vals);
else
    % All valid (3) → use median (scalar)
    rainfall_mm_day_fused = median(valid_vals);
end

== matlab function flood_drainage_system_2_R2025a/Sensor Fusion/Soil Moisture Probe1 ==
  data: moisture_percent output; moisture_scope output; V_scope output; sliderInput input; secondsCounter input; dayCounter input; moisture_type_instring output; Out_voltage output
function [moisture_percent, moisture_scope, V_scope, moisture_type_instring, Out_voltage] = ...
          soilMoistureProbe(sliderInput, secondsCounter, dayCounter)

infil_eff = 0.7;       % infiltration efficiency
d = 300;               % soil depth (mm)
ET_day = 2;            % evapotranspiration loss (mm/day)
ET_rate = ET_day / 86400; % mm/s

persistent VWC prevSec prevDay moisture_scope_last moisture_type_last V_scope_last
if isempty(VWC), VWC = 0; end
if isempty(prevSec), prevSec = 0; end
if isempty(prevDay), prevDay = 0; end
if isempty(moisture_scope_last), moisture_scope_last = 0; end
if isempty(moisture_type_last), moisture_type_last = ""; end
if isempty(V_scope_last), V_scope_last = 0; end

% deltaT (seconds since last tick)
deltaT = secondsCounter - prevSec;
if deltaT <= 0
    deltaT = 1;
end

% rainfall over deltaT (per sec)
rain_mm = sliderInput * deltaT;          % mm of rain in deltaT (per sec)
infil_mm = infil_eff * rain_mm;          % effective infiltration
rain_frac = infil_mm / d;                % fraction of saturation

% ET contribution over deltaT
ET_mm = ET_rate * deltaT;                % mm lost in deltaT
ET_frac = ET_mm / d;                     % fraction of saturation

% Update cumulative Volume Water Concentration (VWC) in fraction
VWC = VWC + rain_frac - ET_frac;
moisture_scope = VWC * 100;

% keep between 0 to 100 only
moisture_scope = max(0, min(100, moisture_scope));
VWC = moisture_scope / 100; 

% classification
if  moisture_scope < 10 % 30
    moisture_type = "Dry";
elseif moisture_scope < 20 % 60
    moisture_type = "Moderate";
elseif moisture_scope < 30 % 90
    moisture_type = "Wet";
else
    moisture_type = "Saturated";
end

% voltage output
V_scope = 0.5 + (moisture_scope/100);

% reset logic (daily rollover)
if double(dayCounter) ~= double(prevDay)
    moisture_scope_last = moisture_scope;
    moisture_type_last = moisture_type;
    V_scope_last = V_scope;

    % carry forward baseline
    VWC = moisture_scope / 100;
    prevDay = double(dayCounter);
end

% update state
prevSec = secondsCounter;

% outputs
moisture_percent = moisture_scope_last;
moisture_type_instring = moisture_type_last;
Out_voltage = V_scope_last;

== matlab function flood_drainage_system_2_R2025a/Sensor Fusion/Soil Moisture Probe2 ==
  data: moisture_percent output; moisture_scope output; V_scope output; sliderInput input; secondsCounter input; dayCounter input; moisture_type_instring output; Out_voltage output
function [moisture_percent, moisture_scope, V_scope, moisture_type_instring, Out_voltage] = ...
          soilMoistureProbe(sliderInput, secondsCounter, dayCounter)

infil_eff = 0.7;       % infiltration efficiency
d = 300;               % soil depth (mm)
ET_day = 2;            % evapotranspiration loss (mm/day)
ET_rate = ET_day / 86400; % mm/s

persistent VWC prevSec prevDay moisture_scope_last moisture_type_last V_scope_last
if isempty(VWC), VWC = 0; end
if isempty(prevSec), prevSec = 0; end
if isempty(prevDay), prevDay = 0; end
if isempty(moisture_scope_last), moisture_scope_last = 0; end
if isempty(moisture_type_last), moisture_type_last = ""; end
if isempty(V_scope_last), V_scope_last = 0; end

% deltaT (seconds since last tick)
deltaT = secondsCounter - prevSec;
if deltaT <= 0
    deltaT = 1;
end

% rainfall over deltaT (per sec)
rain_mm = sliderInput * deltaT;          % mm of rain in deltaT (per sec)
infil_mm = infil_eff * rain_mm;          % effective infiltration
rain_frac = infil_mm / d;                % fraction of saturation

% ET contribution over deltaT
ET_mm = ET_rate * deltaT;                % mm lost in deltaT
ET_frac = ET_mm / d;                     % fraction of saturation

% Update cumulative Volume Water Concentration (VWC) in fraction
VWC = VWC + rain_frac - ET_frac;
moisture_scope = VWC * 100;

% keep between 0 to 100 only
moisture_scope = max(0, min(100, moisture_scope));
VWC = moisture_scope / 100; 

% classification
if  moisture_scope < 10 % 30
    moisture_type = "Dry";
elseif moisture_scope < 20 % 60
    moisture_type = "Moderate";
elseif moisture_scope < 30 % 90
    moisture_type = "Wet";
else
    moisture_type = "Saturated";
end

% voltage output
V_scope = 0.5 + (moisture_scope/100);

% reset logic (daily rollover)
if double(dayCounter) ~= double(prevDay)
    moisture_scope_last = moisture_scope;
    moisture_type_last = moisture_type;
    V_scope_last = V_scope;

    % carry forward baseline
    VWC = moisture_scope / 100;
    prevDay = double(dayCounter);
end

% update state
prevSec = secondsCounter;

% outputs
moisture_percent = moisture_scope_last;
moisture_type_instring = moisture_type_last;
Out_voltage = V_scope_last;

== matlab function flood_drainage_system_2_R2025a/Sensor Fusion/MATLAB Function9 ==
  data: noisy_input input; x_est output
function x_est = kalmanFilter(noisy_input)

persistent x P
if isempty(x), x = noisy_input; end
if isempty(P), P = 1; end


Q = 1e-3;   % process noise covariance
R = 1e-4;   % measurement noise covariance

% prediction
x_pred = x;
P_pred = P + Q;

% update
K = P_pred / (P_pred + R);
x = x_pred + K*(noisy_input - x_pred);
P = (1 - K)*P_pred;

x_est = x;

== matlab function flood_drainage_system_2_R2025a/Sensor Fusion/MATLAB Function10 ==
  data: noisy_input input; x_est output
function x_est = kalmanFilter(noisy_input)

persistent x P
if isempty(x), x = noisy_input; end
if isempty(P), P = 1; end


Q = 1e-3;   % process noise covariance
R = 1e-4;   % measurement noise covariance

% prediction
x_pred = x;
P_pred = P + Q;

% update
K = P_pred / (P_pred + R);
x = x_pred + K*(noisy_input - x_pred);
P = (1 - K)*P_pred;

x_est = x;

== stateflow chart flood_drainage_system_2_R2025a/Sensor Fusion/Tipping Bucket 3 ==
  state Collecting
    during:
    [accumulation, tipCounter, rainfall_scope] = bucketMath(sliderInput, secondsCounter);
  state Reset_Signal
    entry:
    rainfall_mm_per_day = rainfall_scope;
    totaltipCounter = tipCounter;
    tipCounter = 0;
    accumulation = 0;
    rainfall_scope = 0;
  (default) -> Collecting
  Reset_Signal -> Collecting
  Collecting -> Reset_Signal : [Reset == 1]
  data: sliderInput function_input; accumulation function_output; tipCounter function_output; rainfall_scope function_output; secondsCounter function_input; totaltipCounter output; rainfall_scope output; sliderInput input; accumulation local; secondsCounter input; Reset input; rainfall_mm_per_day output; tipCounter local
  function [accumulation, tipCounter, rainfall_scope] = bucketMath(sliderInput, secondsCounter):
    | function [accumulation, tipCounter, rainfall_scope] = bucketMath(sliderInput, secondsCounter)
    | persistent acc tips prevSec
    | if isempty(acc), acc = 0; end
    | if isempty(tips), tips = 0; end
    | if isempty(prevSec), prevSec = 0; end
    | 
    | deltaT = secondsCounter - prevSec;
    | if deltaT <= 0, deltaT = 1; end
    | 
    | acc = acc + sliderInput * deltaT;
    | if acc >= 0.2
    |     tips = tips + 1;
    |     acc = acc - 0.2;
    | end
    | 
    | rainfall_scope = tips * 0.2;
    | prevSec = secondsCounter;
    | 
    | accumulation = acc;
    | tipCounter = tips;

== matlab function flood_drainage_system_2_R2025a/Sensor Fusion/MATLAB Function12 ==
  data: r1 input; moisture_pct_fused output; r2 input; r3 input; fault_flags output
function [moisture_pct_fused, fault_flags] = fuseSoilMoistSensors(r1, r2, r3)
% r1, r2, r3 = filtered outputs from 3 sensor chains
% moisture_pct_fused = fused river elevation signal (scalar double)
% fault_flags = [f1 f2 f3], 1 if sensor flagged faulty

% Parameters
tol = 0.13; % 13% tolerance

% Step 1: Compute mean
vals = [r1 r2 r3];
mean_val = mean(vals);

% Step 2: Fault detection
fault_flags = abs(vals - mean_val) > tol*mean_val;

% Step 3: Fuse valid sensors
valid_vals = vals(~fault_flags);

if isempty(valid_vals)
    % All faulty → fallback to mean
    moisture_pct_fused = mean_val;
elseif isscalar(valid_vals)
    % Only one valid → use it directly (scalar)
    moisture_pct_fused = valid_vals(1);
elseif numel(valid_vals) == 2
    % Two valid → average them (scalar)
    moisture_pct_fused = mean(valid_vals);
else
    % All valid (3) → use median (scalar)
    moisture_pct_fused = median(valid_vals);
end

== matlab function flood_drainage_system_2_R2025a/Sensor Fusion/MATLAB Function13 ==
  data: r1 input; output_voltage_fused output; r2 input; r3 input; fault_flags output
function [output_voltage_fused, fault_flags] = fuseOutputVoltage(r1, r2, r3)
% r1, r2, r3 = filtered outputs from 3 sensor chains
% output_voltage_fused = fused river elevation signal (scalar double)
% fault_flags = [f1 f2 f3], 1 if sensor flagged faulty

% Parameters
tol = 0.05; % 13% tolerance

% Step 1: Compute mean
vals = [r1 r2 r3];
mean_val = mean(vals);

% Step 2: Fault detection
fault_flags = abs(vals - mean_val) > tol*mean_val;

% Step 3: Fuse valid sensors
valid_vals = vals(~fault_flags);

if isempty(valid_vals)
    % All faulty → fallback to mean
    output_voltage_fused = mean_val;
elseif isscalar(valid_vals)
    % Only one valid → use it directly (scalar)
    output_voltage_fused = valid_vals(1);
elseif numel(valid_vals) == 2
    % Two valid → average them (scalar)
    output_voltage_fused = mean(valid_vals);
else
    % All valid (3) → use median (scalar)
    output_voltage_fused = median(valid_vals);
end

== matlab function flood_drainage_system_2_R2025a/Sensor Fusion/MATLAB Function15 ==
  data: noisy_input input; x_est output
function x_est = kalmanFilter(noisy_input)

persistent x P
if isempty(x), x = noisy_input; end
if isempty(P), P = 1; end


Q = 1e-3;   % process noise covariance
R = 1e-4;   % measurement noise covariance

% prediction
x_pred = x;
P_pred = P + Q;

% update
K = P_pred / (P_pred + R);
x = x_pred + K*(noisy_input - x_pred);
P = (1 - K)*P_pred;

x_est = x;

== matlab function flood_drainage_system_2_R2025a/Sensor Fusion/MATLAB Function1 ==
  data: noisy_input input; x_est output
function x_est = kalmanFilter(noisy_input)

persistent x P
if isempty(x), x = noisy_input; end
if isempty(P), P = 1; end


Q = 1e-3;   % process noise covariance
R = 1e-4;   % measurement noise covariance

% prediction
x_pred = x;
P_pred = P + Q;

% update
K = P_pred / (P_pred + R);
x = x_pred + K*(noisy_input - x_pred);
P = (1 - K)*P_pred;

x_est = x;

== matlab function flood_drainage_system_2_R2025a/Sensor Fusion/MATLAB Function14 ==
  data: noisy_input input; x_est output
function x_est = kalmanFilter(noisy_input)

persistent x P
if isempty(x), x = noisy_input; end
if isempty(P), P = 1; end


Q = 1e-3;   % process noise covariance
R = 1e-4;   % measurement noise covariance

% prediction
x_pred = x;
P_pred = P + Q;

% update
K = P_pred / (P_pred + R);
x = x_pred + K*(noisy_input - x_pred);
P = (1 - K)*P_pred;

x_est = x;

== stateflow chart flood_drainage_system_2_R2025a/Rule Based Flood Controller/Water Pump and Sluice Gate Controller ==
  state AUTO_MODE
    entry:
    controlMode=0;
    state NORMAL
      entry:
      PumpCmd=0;
      GateCmd=0;
      Auto_SirenCmd=false;
    state AI_EARLY_MITIGATION
      entry:
      AI_EarlyMitigationActive=1;
      during:
      controlMode = 0;
      PumpCmd = 0;
      GateCmd = 0;
      Auto_SirenCmd = false;
      if Rainfall_Norm >= 0.8 && RiverLevel_Norm >= 0.8
      PumpCmd = 1;
      GateCmd = 1;
      elseif Rainfall_Norm >= RiverLevel_Norm
      PumpCmd = 1;
      else
      GateCmd = 1;
      end
      exit:
      AI_EarlyMitigationActive=0;
    state ALERT
      during:
      PumpCmd = 0;
      GateCmd = 0;
      Auto_SirenCmd = false;
      if Flood_Type == 1
      GateCmd = 1;      % 30%
      elseif Flood_Type == 2
      PumpCmd = 1;      % 30%
      elseif Flood_Type == 3
      PumpCmd = 1;      % 30%
      GateCmd = 1;      % 30%
      end
    state WARNING
      during:
      PumpCmd = 0;
      GateCmd = 0;
      Auto_SirenCmd = false;
      if Flood_Type == 1
      GateCmd = 2;      % 70%
      elseif Flood_Type == 2
      PumpCmd = 2;      % 70%
      elseif Flood_Type == 3
      PumpCmd = 2;      % 70%
      GateCmd = 2;      % 70%
      end
    state DANGER
      entry:
      PumpCmd = 3;          % 100%
      GateCmd = 3;          % 100%
      Auto_SirenCmd = true;
    (default) -> NORMAL
    AI_EARLY_MITIGATION -> NORMAL [order 1] : [AI_FloodFlag == 0 || Confidence <= 0.3]
    NORMAL -> AI_EARLY_MITIGATION [order 2] : [FRI < 0.3 && AI_FloodFlag==1&&Confidence>0.61]
    ALERT -> NORMAL [order 2] : [FRI < 0.29]
    NORMAL -> ALERT [order 1] : [FRI >= 0.3]
    AI_EARLY_MITIGATION -> ALERT [order 2] : [FRI >= 0.3]
    WARNING -> ALERT [order 2] : [FRI < 0.56]
    ALERT -> WARNING [order 1] : [FRI >= 0.6]
    DANGER -> WARNING : [FRI <= 0.76]
    WARNING -> DANGER [order 1] : [FRI >= 0.8]
  state MANUAL_MODE
    state MANUAL_MODE
      during:
      controlMode = 1;
      PumpCmd = Manual_PumpLevel;
      GateCmd = Manual_GateLevel;
      if Manual_PumpLevel > 3
      PumpCmd = 0;
      else
      PumpCmd = Manual_PumpLevel;
      end
      if Manual_GateLevel > 3
      GateCmd = 0;
      else
      GateCmd = Manual_GateLevel;
      end
    (default) -> MANUAL_MODE.MANUAL_MODE
  (default) -> AUTO_MODE
  AUTO_MODE -> MANUAL_MODE : [Manual_Enable==1]
  MANUAL_MODE -> AUTO_MODE : [Manual_Enable==0]
  data: FRI input; Flood_Type input; PumpCmd output; GateCmd output; Auto_SirenCmd output; Manual_Enable input; controlMode output; Manual_GateLevel input; Manual_PumpLevel input; AI_FloodFlag input; Confidence input; AI_EarlyMitigationActive output; Rainfall_Norm input; RiverLevel_Norm input
